simulink model "Project6"  (R2014a)
settings: Solver=ode45  StartTime=0.0  StopTime=310  RelTol=1e-3
undefined symbols (not defined in the file or in its folder): AXI4, Lite
libraries: xbsIndex_r4 x267
(part 2 of 2)

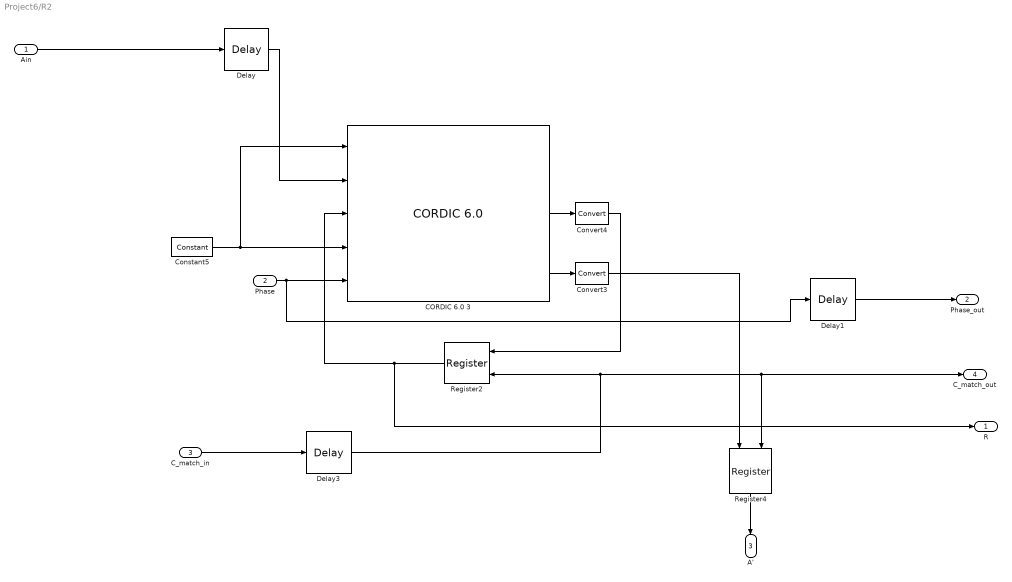
== system Project6/R2 ==
  Ain : Inport
  Phase : Inport  Port=2
  C_match_in : Inport  Port=3
  CORDIC 6.0 3 : xbsIndex_r4/CORDIC 6.0   functional_selection=Rotate  architectural_configuration=Parallel  pipelining_mode=Maximum  data_format=SignedFraction  phase_format=Radians  input_width=16  output_width=16  round_mode=Truncate  iterations=16  precision=16  compensation_scaling=LUT_based  coarse_rotation=on  aclken=off  aresetn=off  out_tready=off  cartesian_has_tuser=off  cartesian_has_tlast=off  cartesian_tuser_width=1  phase_has_tuser=off  phase_has_tlast=off  phase_tuser_width=1  out_tlast_behv=Null  flow_control=NonBlocking  optimize_goal=Performance  trim_axipin_name=on  ip_name=CORDIC  ip_version=6.0  dsptool_ready=true  ipcore_usecache=true  ipcore_useipmodelcache=true  wrapper_available=true  port_translation_map={ 'aclken' => 'en', 'aresetn' => 'rst' }  block_type=cordic_v6_0
      settings: infoedit=CORDIC 6.0
  Constant5 : xbsIndex_r4/Constant  const=1  gui_display_data_type=Boolean  arith_type=Boolean  n_bits=16  bin_pt=14  preci_type=Single  exp_width=8  frac_width=24  explicit_period=on  period=1  equ=P=C  opselect=C  inp2=PCIN>>17  opr=+  inp1=P  carry=CIN  dbl_ovrd=off  block_type=constant
  Convert3 : xbsIndex_r4/Convert  gui_display_data_type=Fixed-point  arith_type="Signed  (2's comp)"  n_bits=16  bin_pt=14  float_type=Single  exp_bits=8  fraction_bits=24  quantization=Truncate  overflow=Wrap  en=off  latency=0  pipeline=on  dbl_ovrd=off  block_type=convert
  Convert4 : xbsIndex_r4/Convert  gui_display_data_type=Fixed-point  arith_type="Signed  (2's comp)"  n_bits=16  bin_pt=14  float_type=Single  exp_bits=8  fraction_bits=24  quantization=Truncate  overflow=Wrap  en=off  latency=0  pipeline=on  dbl_ovrd=off  block_type=convert
  Delay : xbsIndex_r4/Delay  rst=off  infoeditControl=Selection of Reset will increase slice count due to use of real FFs and instead of SRLs  en=off  latency=22  reg_retiming=off  dbl_ovrd=off  block_type=delay
  Delay1 : xbsIndex_r4/Delay  rst=off  infoeditControl=Selection of Reset will increase slice count due to use of real FFs and instead of SRLs  en=off  latency=1  reg_retiming=off  dbl_ovrd=off  block_type=delay
  Delay3 : xbsIndex_r4/Delay  rst=off  infoeditControl=Selection of Reset will increase slice count due to use of real FFs and instead of SRLs  en=off  latency=1  reg_retiming=off  dbl_ovrd=off  block_type=delay
  Register2 : xbsIndex_r4/Register  init=0  rst=off  en=on  dbl_ovrd=off  block_type=register
  Register4 : xbsIndex_r4/Register  init=0  rst=off  en=on  dbl_ovrd=off  block_type=register
  R : Outport
  Phase_out : Outport  Port=2
  A' : Outport  Port=3
  C_match_out : Outport  Port=4
  wires:
  Ain/1 -> Delay/1
  Delay/1 -> CORDIC 6.0 3/2
  Convert4/1 -> Register2/1
  CORDIC 6.0 3/2 -> Convert4/1
  Register2/1 -> R/1, CORDIC 6.0 3/3
  CORDIC 6.0 3/3 -> Convert3/1
  Constant5/1 -> CORDIC 6.0 3/1, CORDIC 6.0 3/4
  Register4/1 -> A'/1
  Convert3/1 -> Register4/1
  Phase/1 -> Delay1/1, CORDIC 6.0 3/5
  Delay3/1 -> Register2/2, C_match_out/1, Register4/2
  C_match_in/1 -> Delay3/1
  Delay1/1 -> Phase_out/1

== system Project6/R22 ==
  Ain : Inport
  "C_match_in " : Inport  Port=2
  CORDIC 6.0 1 : xbsIndex_r4/CORDIC 6.0   functional_selection=Rotate  architectural_configuration=Parallel  pipelining_mode=Maximum  data_format=SignedFraction  phase_format=Radians  input_width=16  output_width=16  round_mode=Truncate  iterations=16  precision=16  compensation_scaling=LUT_based  coarse_rotation=on  aclken=off  aresetn=off  out_tready=off  cartesian_has_tuser=off  cartesian_has_tlast=off  cartesian_tuser_width=1  phase_has_tuser=off  phase_has_tlast=off  phase_tuser_width=1  out_tlast_behv=Null  flow_control=NonBlocking  optimize_goal=Performance  trim_axipin_name=on  ip_name=CORDIC  ip_version=6.0  dsptool_ready=true  ipcore_usecache=true  ipcore_useipmodelcache=true  wrapper_available=true  port_translation_map={ 'aclken' => 'en', 'aresetn' => 'rst' }  block_type=cordic_v6_0
      settings: infoedit=CORDIC 6.0
  CORDIC 6.0 2 : xbsIndex_r4/CORDIC 6.0   functional_selection=Arc_Tan  architectural_configuration=Parallel  pipelining_mode=Maximum  data_format=SignedFraction  phase_format=Radians  input_width=16  output_width=16  round_mode=Truncate  iterations=16  precision=16  compensation_scaling=No_Scale_Compensation  coarse_rotation=on  aclken=off  aresetn=off  out_tready=off  cartesian_has_tuser=off  cartesian_has_tlast=off  cartesian_tuser_width=1  phase_has_tuser=off  phase_has_tlast=off  phase_tuser_width=1  out_tlast_behv=Null  flow_control=NonBlocking  optimize_goal=Performance  trim_axipin_name=on  ip_name=CORDIC  ip_version=6.0  dsptool_ready=true  ipcore_usecache=true  ipcore_useipmodelcache=true  wrapper_available=true  port_translation_map={ 'aclken' => 'en', 'aresetn' => 'rst' }  block_type=cordic_v6_0
      settings: infoedit=CORDIC 6.0
  Constant1 : xbsIndex_r4/Constant  const=1  gui_display_data_type=Boolean  arith_type=Boolean  n_bits=16  bin_pt=14  preci_type=Single  exp_width=8  frac_width=24  explicit_period=on  period=1  equ=P=C  opselect=C  inp2=PCIN>>17  opr=+  inp1=P  carry=CIN  dbl_ovrd=off  block_type=constant
  Constant2 : xbsIndex_r4/Constant  const=1  gui_display_data_type=Boolean  arith_type=Boolean  n_bits=16  bin_pt=14  preci_type=Single  exp_width=8  frac_width=24  explicit_period=on  period=1  equ=P=C  opselect=C  inp2=PCIN>>17  opr=+  inp1=P  carry=CIN  dbl_ovrd=off  block_type=constant
  Convert1 : xbsIndex_r4/Convert  gui_display_data_type=Fixed-point  arith_type="Signed  (2's comp)"  n_bits=16  bin_pt=14  float_type=Single  exp_bits=8  fraction_bits=24  quantization=Truncate  overflow=Wrap  en=off  latency=0  pipeline=on  dbl_ovrd=off  block_type=convert
  Convert2 : xbsIndex_r4/Convert  gui_display_data_type=Fixed-point  arith_type="Signed  (2's comp)"  n_bits=16  bin_pt=14  float_type=Single  exp_bits=8  fraction_bits=24  quantization=Truncate  overflow=Wrap  en=off  latency=0  pipeline=on  dbl_ovrd=off  block_type=convert
  Delay1 : xbsIndex_r4/Delay  rst=off  infoeditControl=Selection of Reset will increase slice count due to use of real FFs and instead of SRLs  en=off  latency=1  reg_retiming=off  dbl_ovrd=off  block_type=delay
  Register : xbsIndex_r4/Register  init=0  rst=off  en=on  dbl_ovrd=off  block_type=register
  Scope1 : Scope  NumInputPorts=2
      settings: YMin=-5~-5  YMax=5~5  SaveName=ScopeData5
  Phase : Outport
  C_match_out : Outport  Port=2
  R : Outport  Port=3
  wires:
  Constant1/1 -> CORDIC 6.0 1/1, CORDIC 6.0 1/4
  Constant2/1 -> CORDIC 6.0 2/1
  Delay1/1 -> Phase/1
  CORDIC 6.0 1/2 -> Convert2/1
  CORDIC 6.0 2/2 -> Delay1/1, CORDIC 6.0 1/5
  Ain/1 -> CORDIC 6.0 2/3, Scope1/1, CORDIC 6.0 1/2
  Register/1 -> R/1, Convert1/1, CORDIC 6.0 1/3
  Convert2/1 -> Register/1
  "C_match_in "/1 -> Register/2, C_match_out/1
  Convert1/1 -> Scope1/2, CORDIC 6.0 2/2

== system Project6/R23 ==
  Ain : Inport
  Phase : Inport  Port=2
  C_match_in : Inport  Port=3
  CORDIC 6.0 3 : xbsIndex_r4/CORDIC 6.0   functional_selection=Rotate  architectural_configuration=Parallel  pipelining_mode=Maximum  data_format=SignedFraction  phase_format=Radians  input_width=16  output_width=16  round_mode=Truncate  iterations=16  precision=16  compensation_scaling=LUT_based  coarse_rotation=on  aclken=off  aresetn=off  out_tready=off  cartesian_has_tuser=off  cartesian_has_tlast=off  cartesian_tuser_width=1  phase_has_tuser=off  phase_has_tlast=off  phase_tuser_width=1  out_tlast_behv=Null  flow_control=NonBlocking  optimize_goal=Performance  trim_axipin_name=on  ip_name=CORDIC  ip_version=6.0  dsptool_ready=true  ipcore_usecache=true  ipcore_useipmodelcache=true  wrapper_available=true  port_translation_map={ 'aclken' => 'en', 'aresetn' => 'rst' }  block_type=cordic_v6_0
      settings: infoedit=CORDIC 6.0
  Constant5 : xbsIndex_r4/Constant  const=1  gui_display_data_type=Boolean  arith_type=Boolean  n_bits=16  bin_pt=14  preci_type=Single  exp_width=8  frac_width=24  explicit_period=on  period=1  equ=P=C  opselect=C  inp2=PCIN>>17  opr=+  inp1=P  carry=CIN  dbl_ovrd=off  block_type=constant
  Convert3 : xbsIndex_r4/Convert  gui_display_data_type=Fixed-point  arith_type="Signed  (2's comp)"  n_bits=16  bin_pt=14  float_type=Single  exp_bits=8  fraction_bits=24  quantization=Truncate  overflow=Wrap  en=off  latency=0  pipeline=on  dbl_ovrd=off  block_type=convert
  Convert4 : xbsIndex_r4/Convert  gui_display_data_type=Fixed-point  arith_type="Signed  (2's comp)"  n_bits=16  bin_pt=14  float_type=Single  exp_bits=8  fraction_bits=24  quantization=Truncate  overflow=Wrap  en=off  latency=0  pipeline=on  dbl_ovrd=off  block_type=convert
  Delay1 : xbsIndex_r4/Delay  rst=off  infoeditControl=Selection of Reset will increase slice count due to use of real FFs and instead of SRLs  en=off  latency=1  reg_retiming=off  dbl_ovrd=off  block_type=delay
  Delay2 : xbsIndex_r4/Delay  rst=off  infoeditControl=Selection of Reset will increase slice count due to use of real FFs and instead of SRLs  en=off  latency=22  reg_retiming=off  dbl_ovrd=off  block_type=delay
  Delay3 : xbsIndex_r4/Delay  rst=off  infoeditControl=Selection of Reset will increase slice count due to use of real FFs and instead of SRLs  en=off  latency=1  reg_retiming=off  dbl_ovrd=off  block_type=delay
  Register2 : xbsIndex_r4/Register  init=0  rst=off  en=on  dbl_ovrd=off  block_type=register
  Register4 : xbsIndex_r4/Register  init=0  rst=off  en=on  dbl_ovrd=off  block_type=register
  R : Outport
  Phase_out : Outport  Port=2
  A' : Outport  Port=3
  C_match_out : Outport  Port=4
  wires:
  CORDIC 6.0 3/2 -> Convert4/1
  Register2/1 -> R/1, CORDIC 6.0 3/3
  CORDIC 6.0 3/3 -> Convert3/1
  Constant5/1 -> CORDIC 6.0 3/1, CORDIC 6.0 3/4
  Register4/1 -> A'/1
  Convert3/1 -> Register4/1
  Delay3/1 -> Register2/2, C_match_out/1, Register4/2
  C_match_in/1 -> Delay3/1
  Delay1/1 -> Phase_out/1
  Ain/1 -> Delay2/1
  Phase/1 -> CORDIC 6.0 3/5, Delay1/1
  Delay2/1 -> CORDIC 6.0 3/2
  Convert4/1 -> Register2/1

== system Project6/R24 ==
  Ain : Inport
  Phase : Inport  Port=2
  C_match_in : Inport  Port=3
  CORDIC 6.0 3 : xbsIndex_r4/CORDIC 6.0   functional_selection=Rotate  architectural_configuration=Parallel  pipelining_mode=Maximum  data_format=SignedFraction  phase_format=Radians  input_width=16  output_width=16  round_mode=Truncate  iterations=16  precision=16  compensation_scaling=LUT_based  coarse_rotation=on  aclken=off  aresetn=off  out_tready=off  cartesian_has_tuser=off  cartesian_has_tlast=off  cartesian_tuser_width=1  phase_has_tuser=off  phase_has_tlast=off  phase_tuser_width=1  out_tlast_behv=Null  flow_control=NonBlocking  optimize_goal=Performance  trim_axipin_name=on  ip_name=CORDIC  ip_version=6.0  dsptool_ready=true  ipcore_usecache=true  ipcore_useipmodelcache=true  wrapper_available=true  port_translation_map={ 'aclken' => 'en', 'aresetn' => 'rst' }  block_type=cordic_v6_0
      settings: infoedit=CORDIC 6.0
  Constant5 : xbsIndex_r4/Constant  const=1  gui_display_data_type=Boolean  arith_type=Boolean  n_bits=16  bin_pt=14  preci_type=Single  exp_width=8  frac_width=24  explicit_period=on  period=1  equ=P=C  opselect=C  inp2=PCIN>>17  opr=+  inp1=P  carry=CIN  dbl_ovrd=off  block_type=constant
  Convert3 : xbsIndex_r4/Convert  gui_display_data_type=Fixed-point  arith_type="Signed  (2's comp)"  n_bits=16  bin_pt=14  float_type=Single  exp_bits=8  fraction_bits=24  quantization=Truncate  overflow=Wrap  en=off  latency=0  pipeline=on  dbl_ovrd=off  block_type=convert
  Convert4 : xbsIndex_r4/Convert  gui_display_data_type=Fixed-point  arith_type="Signed  (2's comp)"  n_bits=16  bin_pt=14  float_type=Single  exp_bits=8  fraction_bits=24  quantization=Truncate  overflow=Wrap  en=off  latency=0  pipeline=on  dbl_ovrd=off  block_type=convert
  Delay : xbsIndex_r4/Delay  rst=off  infoeditControl=Selection of Reset will increase slice count due to use of real FFs and instead of SRLs  en=off  latency=22  reg_retiming=off  dbl_ovrd=off  block_type=delay
  Delay1 : xbsIndex_r4/Delay  rst=off  infoeditControl=Selection of Reset will increase slice count due to use of real FFs and instead of SRLs  en=off  latency=1  reg_retiming=off  dbl_ovrd=off  block_type=delay
  Delay3 : xbsIndex_r4/Delay  rst=off  infoeditControl=Selection of Reset will increase slice count due to use of real FFs and instead of SRLs  en=off  latency=1  reg_retiming=off  dbl_ovrd=off  block_type=delay
  Register2 : xbsIndex_r4/Register  init=0  rst=off  en=on  dbl_ovrd=off  block_type=register
  Register4 : xbsIndex_r4/Register  init=0  rst=off  en=on  dbl_ovrd=off  block_type=register
  R : Outport
  Phase_out : Outport  Port=2
  A' : Outport  Port=3
  C_match_out : Outport  Port=4
  wires:
  Ain/1 -> Delay/1
  Delay/1 -> CORDIC 6.0 3/2
  Convert4/1 -> Register2/1
  CORDIC 6.0 3/2 -> Convert4/1
  Register2/1 -> R/1, CORDIC 6.0 3/3
  CORDIC 6.0 3/3 -> Convert3/1
  Constant5/1 -> CORDIC 6.0 3/1, CORDIC 6.0 3/4
  Register4/1 -> A'/1
  Convert3/1 -> Register4/1
  Phase/1 -> Delay1/1, CORDIC 6.0 3/5
  Delay3/1 -> Register2/2, C_match_out/1, Register4/2
  C_match_in/1 -> Delay3/1
  Delay1/1 -> Phase_out/1

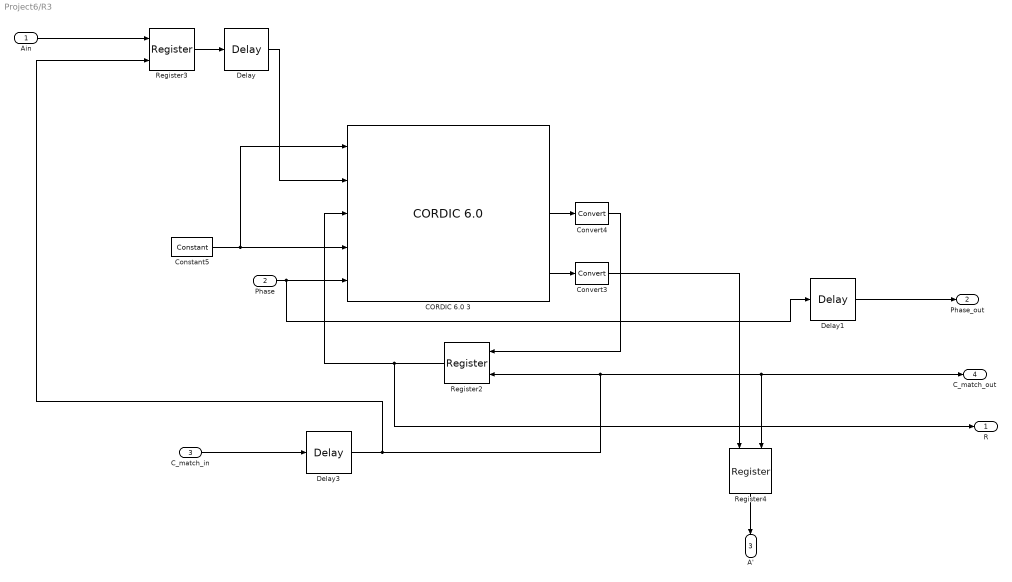
== system Project6/R3 ==
  Ain : Inport
  Phase : Inport  Port=2
  C_match_in : Inport  Port=3
  CORDIC 6.0 3 : xbsIndex_r4/CORDIC 6.0   functional_selection=Rotate  architectural_configuration=Parallel  pipelining_mode=Maximum  data_format=SignedFraction  phase_format=Radians  input_width=16  output_width=16  round_mode=Truncate  iterations=16  precision=16  compensation_scaling=LUT_based  coarse_rotation=on  aclken=off  aresetn=off  out_tready=off  cartesian_has_tuser=off  cartesian_has_tlast=off  cartesian_tuser_width=1  phase_has_tuser=off  phase_has_tlast=off  phase_tuser_width=1  out_tlast_behv=Null  flow_control=NonBlocking  optimize_goal=Performance  trim_axipin_name=on  ip_name=CORDIC  ip_version=6.0  dsptool_ready=true  ipcore_usecache=true  ipcore_useipmodelcache=true  wrapper_available=true  port_translation_map={ 'aclken' => 'en', 'aresetn' => 'rst' }  block_type=cordic_v6_0
      settings: infoedit=CORDIC 6.0
  Constant5 : xbsIndex_r4/Constant  const=1  gui_display_data_type=Boolean  arith_type=Boolean  n_bits=16  bin_pt=14  preci_type=Single  exp_width=8  frac_width=24  explicit_period=on  period=1  equ=P=C  opselect=C  inp2=PCIN>>17  opr=+  inp1=P  carry=CIN  dbl_ovrd=off  block_type=constant
  Convert3 : xbsIndex_r4/Convert  gui_display_data_type=Fixed-point  arith_type="Signed  (2's comp)"  n_bits=16  bin_pt=14  float_type=Single  exp_bits=8  fraction_bits=24  quantization=Truncate  overflow=Wrap  en=off  latency=0  pipeline=on  dbl_ovrd=off  block_type=convert
  Convert4 : xbsIndex_r4/Convert  gui_display_data_type=Fixed-point  arith_type="Signed  (2's comp)"  n_bits=16  bin_pt=14  float_type=Single  exp_bits=8  fraction_bits=24  quantization=Truncate  overflow=Wrap  en=off  latency=0  pipeline=on  dbl_ovrd=off  block_type=convert
  Delay : xbsIndex_r4/Delay  rst=off  infoeditControl=Selection of Reset will increase slice count due to use of real FFs and instead of SRLs  en=off  latency=22  reg_retiming=off  dbl_ovrd=off  block_type=delay
  Delay1 : xbsIndex_r4/Delay  rst=off  infoeditControl=Selection of Reset will increase slice count due to use of real FFs and instead of SRLs  en=off  latency=1  reg_retiming=off  dbl_ovrd=off  block_type=delay
  Delay3 : xbsIndex_r4/Delay  rst=off  infoeditControl=Selection of Reset will increase slice count due to use of real FFs and instead of SRLs  en=off  latency=1  reg_retiming=off  dbl_ovrd=off  block_type=delay
  Register2 : xbsIndex_r4/Register  init=0  rst=off  en=on  dbl_ovrd=off  block_type=register
  Register3 : xbsIndex_r4/Register  init=0  rst=off  en=on  dbl_ovrd=off  block_type=register
  Register4 : xbsIndex_r4/Register  init=0  rst=off  en=on  dbl_ovrd=off  block_type=register
  R : Outport
  Phase_out : Outport  Port=2
  A' : Outport  Port=3
  C_match_out : Outport  Port=4
  wires:
  Register3/1 -> Delay/1
  Ain/1 -> Register3/1
  Delay/1 -> CORDIC 6.0 3/2
  Convert4/1 -> Register2/1
  CORDIC 6.0 3/2 -> Convert4/1
  Register2/1 -> R/1, CORDIC 6.0 3/3
  CORDIC 6.0 3/3 -> Convert3/1
  Constant5/1 -> CORDIC 6.0 3/1, CORDIC 6.0 3/4
  Register4/1 -> A'/1
  Convert3/1 -> Register4/1
  Phase/1 -> Delay1/1, CORDIC 6.0 3/5
  Delay3/1 -> Register3/2, Register2/2, C_match_out/1, Register4/2
  C_match_in/1 -> Delay3/1
  Delay1/1 -> Phase_out/1

== system Project6/R33 ==
  Ain : Inport
  "C_match_in " : Inport  Port=2
  CORDIC 6.0 1 : xbsIndex_r4/CORDIC 6.0   functional_selection=Rotate  architectural_configuration=Parallel  pipelining_mode=Maximum  data_format=SignedFraction  phase_format=Radians  input_width=16  output_width=16  round_mode=Truncate  iterations=16  precision=16  compensation_scaling=LUT_based  coarse_rotation=on  aclken=off  aresetn=off  out_tready=off  cartesian_has_tuser=off  cartesian_has_tlast=off  cartesian_tuser_width=1  phase_has_tuser=off  phase_has_tlast=off  phase_tuser_width=1  out_tlast_behv=Null  flow_control=NonBlocking  optimize_goal=Performance  trim_axipin_name=on  ip_name=CORDIC  ip_version=6.0  dsptool_ready=true  ipcore_usecache=true  ipcore_useipmodelcache=true  wrapper_available=true  port_translation_map={ 'aclken' => 'en', 'aresetn' => 'rst' }  block_type=cordic_v6_0
      settings: infoedit=CORDIC 6.0
  CORDIC 6.0 2 : xbsIndex_r4/CORDIC 6.0   functional_selection=Arc_Tan  architectural_configuration=Parallel  pipelining_mode=Maximum  data_format=SignedFraction  phase_format=Radians  input_width=16  output_width=16  round_mode=Truncate  iterations=16  precision=16  compensation_scaling=No_Scale_Compensation  coarse_rotation=on  aclken=off  aresetn=off  out_tready=off  cartesian_has_tuser=off  cartesian_has_tlast=off  cartesian_tuser_width=1  phase_has_tuser=off  phase_has_tlast=off  phase_tuser_width=1  out_tlast_behv=Null  flow_control=NonBlocking  optimize_goal=Performance  trim_axipin_name=on  ip_name=CORDIC  ip_version=6.0  dsptool_ready=true  ipcore_usecache=true  ipcore_useipmodelcache=true  wrapper_available=true  port_translation_map={ 'aclken' => 'en', 'aresetn' => 'rst' }  block_type=cordic_v6_0
      settings: infoedit=CORDIC 6.0
  Constant1 : xbsIndex_r4/Constant  const=1  gui_display_data_type=Boolean  arith_type=Boolean  n_bits=16  bin_pt=14  preci_type=Single  exp_width=8  frac_width=24  explicit_period=on  period=1  equ=P=C  opselect=C  inp2=PCIN>>17  opr=+  inp1=P  carry=CIN  dbl_ovrd=off  block_type=constant
  Constant2 : xbsIndex_r4/Constant  const=1  gui_display_data_type=Boolean  arith_type=Boolean  n_bits=16  bin_pt=14  preci_type=Single  exp_width=8  frac_width=24  explicit_period=on  period=1  equ=P=C  opselect=C  inp2=PCIN>>17  opr=+  inp1=P  carry=CIN  dbl_ovrd=off  block_type=constant
  Convert1 : xbsIndex_r4/Convert  gui_display_data_type=Fixed-point  arith_type="Signed  (2's comp)"  n_bits=16  bin_pt=14  float_type=Single  exp_bits=8  fraction_bits=24  quantization=Truncate  overflow=Wrap  en=off  latency=0  pipeline=on  dbl_ovrd=off  block_type=convert
  Convert2 : xbsIndex_r4/Convert  gui_display_data_type=Fixed-point  arith_type="Signed  (2's comp)"  n_bits=16  bin_pt=14  float_type=Single  exp_bits=8  fraction_bits=24  quantization=Truncate  overflow=Wrap  en=off  latency=0  pipeline=on  dbl_ovrd=off  block_type=convert
  Delay1 : xbsIndex_r4/Delay  rst=off  infoeditControl=Selection of Reset will increase slice count due to use of real FFs and instead of SRLs  en=off  latency=1  reg_retiming=off  dbl_ovrd=off  block_type=delay
  Register : xbsIndex_r4/Register  init=0  rst=off  en=on  dbl_ovrd=off  block_type=register
  Phase : Outport
  C_match_out : Outport  Port=2
  R : Outport  Port=3
  wires:
  Constant1/1 -> CORDIC 6.0 1/1, CORDIC 6.0 1/4
  Constant2/1 -> CORDIC 6.0 2/1
  Delay1/1 -> Phase/1
  CORDIC 6.0 1/2 -> Convert2/1
  CORDIC 6.0 2/2 -> Delay1/1, CORDIC 6.0 1/5
  Ain/1 -> CORDIC 6.0 2/3, CORDIC 6.0 1/2
  Convert1/1 -> CORDIC 6.0 2/2
  Register/1 -> R/1, Convert1/1, CORDIC 6.0 1/3
  Convert2/1 -> Register/1
  "C_match_in "/1 -> Register/2, C_match_out/1

== system Project6/R34 ==
  Ain : Inport
  Phase : Inport  Port=2
  C_match_in : Inport  Port=3
  CORDIC 6.0 3 : xbsIndex_r4/CORDIC 6.0   functional_selection=Rotate  architectural_configuration=Parallel  pipelining_mode=Maximum  data_format=SignedFraction  phase_format=Radians  input_width=16  output_width=16  round_mode=Truncate  iterations=16  precision=16  compensation_scaling=LUT_based  coarse_rotation=on  aclken=off  aresetn=off  out_tready=off  cartesian_has_tuser=off  cartesian_has_tlast=off  cartesian_tuser_width=1  phase_has_tuser=off  phase_has_tlast=off  phase_tuser_width=1  out_tlast_behv=Null  flow_control=NonBlocking  optimize_goal=Performance  trim_axipin_name=on  ip_name=CORDIC  ip_version=6.0  dsptool_ready=true  ipcore_usecache=true  ipcore_useipmodelcache=true  wrapper_available=true  port_translation_map={ 'aclken' => 'en', 'aresetn' => 'rst' }  block_type=cordic_v6_0
      settings: infoedit=CORDIC 6.0
  Constant5 : xbsIndex_r4/Constant  const=1  gui_display_data_type=Boolean  arith_type=Boolean  n_bits=16  bin_pt=14  preci_type=Single  exp_width=8  frac_width=24  explicit_period=on  period=1  equ=P=C  opselect=C  inp2=PCIN>>17  opr=+  inp1=P  carry=CIN  dbl_ovrd=off  block_type=constant
  Convert3 : xbsIndex_r4/Convert  gui_display_data_type=Fixed-point  arith_type="Signed  (2's comp)"  n_bits=16  bin_pt=14  float_type=Single  exp_bits=8  fraction_bits=24  quantization=Truncate  overflow=Wrap  en=off  latency=0  pipeline=on  dbl_ovrd=off  block_type=convert
  Convert4 : xbsIndex_r4/Convert  gui_display_data_type=Fixed-point  arith_type="Signed  (2's comp)"  n_bits=16  bin_pt=14  float_type=Single  exp_bits=8  fraction_bits=24  quantization=Truncate  overflow=Wrap  en=off  latency=0  pipeline=on  dbl_ovrd=off  block_type=convert
  Delay : xbsIndex_r4/Delay  rst=off  infoeditControl=Selection of Reset will increase slice count due to use of real FFs and instead of SRLs  en=off  latency=22  reg_retiming=off  dbl_ovrd=off  block_type=delay
  Delay1 : xbsIndex_r4/Delay  rst=off  infoeditControl=Selection of Reset will increase slice count due to use of real FFs and instead of SRLs  en=off  latency=1  reg_retiming=off  dbl_ovrd=off  block_type=delay
  Delay3 : xbsIndex_r4/Delay  rst=off  infoeditControl=Selection of Reset will increase slice count due to use of real FFs and instead of SRLs  en=off  latency=1  reg_retiming=off  dbl_ovrd=off  block_type=delay
  Register2 : xbsIndex_r4/Register  init=0  rst=off  en=on  dbl_ovrd=off  block_type=register
  Register4 : xbsIndex_r4/Register  init=0  rst=off  en=on  dbl_ovrd=off  block_type=register
  R : Outport
  Phase_out : Outport  Port=2
  A' : Outport  Port=3
  C_match_out : Outport  Port=4
  wires:
  Ain/1 -> Delay/1
  Delay/1 -> CORDIC 6.0 3/2
  Convert4/1 -> Register2/1
  CORDIC 6.0 3/2 -> Convert4/1
  Register2/1 -> R/1, CORDIC 6.0 3/3
  CORDIC 6.0 3/3 -> Convert3/1
  Constant5/1 -> CORDIC 6.0 3/1, CORDIC 6.0 3/4
  Register4/1 -> A'/1
  Convert3/1 -> Register4/1
  Phase/1 -> Delay1/1, CORDIC 6.0 3/5
  Delay3/1 -> Register2/2, C_match_out/1, Register4/2
  C_match_in/1 -> Delay3/1
  Delay1/1 -> Phase_out/1

== system Project6/R4 ==
  Ain : Inport
  Phase : Inport  Port=2
  C_match_in : Inport  Port=3
  CORDIC 6.0 3 : xbsIndex_r4/CORDIC 6.0   functional_selection=Rotate  architectural_configuration=Parallel  pipelining_mode=Maximum  data_format=SignedFraction  phase_format=Radians  input_width=16  output_width=16  round_mode=Truncate  iterations=16  precision=16  compensation_scaling=LUT_based  coarse_rotation=on  aclken=off  aresetn=off  out_tready=off  cartesian_has_tuser=off  cartesian_has_tlast=off  cartesian_tuser_width=1  phase_has_tuser=off  phase_has_tlast=off  phase_tuser_width=1  out_tlast_behv=Null  flow_control=NonBlocking  optimize_goal=Performance  trim_axipin_name=on  ip_name=CORDIC  ip_version=6.0  dsptool_ready=true  ipcore_usecache=true  ipcore_useipmodelcache=true  wrapper_available=true  port_translation_map={ 'aclken' => 'en', 'aresetn' => 'rst' }  block_type=cordic_v6_0
      settings: infoedit=CORDIC 6.0
  Constant5 : xbsIndex_r4/Constant  const=1  gui_display_data_type=Boolean  arith_type=Boolean  n_bits=16  bin_pt=14  preci_type=Single  exp_width=8  frac_width=24  explicit_period=on  period=1  equ=P=C  opselect=C  inp2=PCIN>>17  opr=+  inp1=P  carry=CIN  dbl_ovrd=off  block_type=constant
  Convert3 : xbsIndex_r4/Convert  gui_display_data_type=Fixed-point  arith_type="Signed  (2's comp)"  n_bits=16  bin_pt=14  float_type=Single  exp_bits=8  fraction_bits=24  quantization=Truncate  overflow=Wrap  en=off  latency=0  pipeline=on  dbl_ovrd=off  block_type=convert
  Convert4 : xbsIndex_r4/Convert  gui_display_data_type=Fixed-point  arith_type="Signed  (2's comp)"  n_bits=16  bin_pt=14  float_type=Single  exp_bits=8  fraction_bits=24  quantization=Truncate  overflow=Wrap  en=off  latency=0  pipeline=on  dbl_ovrd=off  block_type=convert
  Delay : xbsIndex_r4/Delay  rst=off  infoeditControl=Selection of Reset will increase slice count due to use of real FFs and instead of SRLs  en=off  latency=22  reg_retiming=off  dbl_ovrd=off  block_type=delay
  Delay1 : xbsIndex_r4/Delay  rst=off  infoeditControl=Selection of Reset will increase slice count due to use of real FFs and instead of SRLs  en=off  latency=1  reg_retiming=off  dbl_ovrd=off  block_type=delay
  Delay3 : xbsIndex_r4/Delay  rst=off  infoeditControl=Selection of Reset will increase slice count due to use of real FFs and instead of SRLs  en=off  latency=1  reg_retiming=off  dbl_ovrd=off  block_type=delay
  Register2 : xbsIndex_r4/Register  init=0  rst=off  en=on  dbl_ovrd=off  block_type=register
  Register4 : xbsIndex_r4/Register  init=0  rst=off  en=on  dbl_ovrd=off  block_type=register
  R : Outport
  Phase_out : Outport  Port=2
  A' : Outport  Port=3
  C_match_out : Outport  Port=4
  wires:
  Ain/1 -> Delay/1
  Delay/1 -> CORDIC 6.0 3/2
  Convert4/1 -> Register2/1
  CORDIC 6.0 3/2 -> Convert4/1
  Register2/1 -> R/1, CORDIC 6.0 3/3
  CORDIC 6.0 3/3 -> Convert3/1
  Constant5/1 -> CORDIC 6.0 3/1, CORDIC 6.0 3/4
  Register4/1 -> A'/1
  Convert3/1 -> Register4/1
  Phase/1 -> Delay1/1, CORDIC 6.0 3/5
  Delay3/1 -> Register2/2, C_match_out/1, Register4/2
  C_match_in/1 -> Delay3/1
  Delay1/1 -> Phase_out/1

== system Project6/R5 ==
  Ain : Inport
  Phase : Inport  Port=2
  C_match_in : Inport  Port=3
  CORDIC 6.0 3 : xbsIndex_r4/CORDIC 6.0   functional_selection=Rotate  architectural_configuration=Parallel  pipelining_mode=Maximum  data_format=SignedFraction  phase_format=Radians  input_width=16  output_width=16  round_mode=Truncate  iterations=16  precision=16  compensation_scaling=LUT_based  coarse_rotation=on  aclken=off  aresetn=off  out_tready=off  cartesian_has_tuser=off  cartesian_has_tlast=off  cartesian_tuser_width=1  phase_has_tuser=off  phase_has_tlast=off  phase_tuser_width=1  out_tlast_behv=Null  flow_control=NonBlocking  optimize_goal=Performance  trim_axipin_name=on  ip_name=CORDIC  ip_version=6.0  dsptool_ready=true  ipcore_usecache=true  ipcore_useipmodelcache=true  wrapper_available=true  port_translation_map={ 'aclken' => 'en', 'aresetn' => 'rst' }  block_type=cordic_v6_0
      settings: infoedit=CORDIC 6.0
  Constant5 : xbsIndex_r4/Constant  const=1  gui_display_data_type=Boolean  arith_type=Boolean  n_bits=16  bin_pt=14  preci_type=Single  exp_width=8  frac_width=24  explicit_period=on  period=1  equ=P=C  opselect=C  inp2=PCIN>>17  opr=+  inp1=P  carry=CIN  dbl_ovrd=off  block_type=constant
  Convert3 : xbsIndex_r4/Convert  gui_display_data_type=Fixed-point  arith_type="Signed  (2's comp)"  n_bits=16  bin_pt=14  float_type=Single  exp_bits=8  fraction_bits=24  quantization=Truncate  overflow=Wrap  en=off  latency=0  pipeline=on  dbl_ovrd=off  block_type=convert
  Convert4 : xbsIndex_r4/Convert  gui_display_data_type=Fixed-point  arith_type="Signed  (2's comp)"  n_bits=16  bin_pt=14  float_type=Single  exp_bits=8  fraction_bits=24  quantization=Truncate  overflow=Wrap  en=off  latency=0  pipeline=on  dbl_ovrd=off  block_type=convert
  Delay : xbsIndex_r4/Delay  rst=off  infoeditControl=Selection of Reset will increase slice count due to use of real FFs and instead of SRLs  en=off  latency=22  reg_retiming=off  dbl_ovrd=off  block_type=delay
  Delay1 : xbsIndex_r4/Delay  rst=off  infoeditControl=Selection of Reset will increase slice count due to use of real FFs and instead of SRLs  en=off  latency=1  reg_retiming=off  dbl_ovrd=off  block_type=delay
  Delay3 : xbsIndex_r4/Delay  rst=off  infoeditControl=Selection of Reset will increase slice count due to use of real FFs and instead of SRLs  en=off  latency=1  reg_retiming=off  dbl_ovrd=off  block_type=delay
  Register2 : xbsIndex_r4/Register  init=0  rst=off  en=on  dbl_ovrd=off  block_type=register
  Register4 : xbsIndex_r4/Register  init=0  rst=off  en=on  dbl_ovrd=off  block_type=register
  R : Outport
  Phase_out : Outport  Port=2
  A' : Outport  Port=3
  C_match_out : Outport  Port=4
  wires:
  Ain/1 -> Delay/1
  Delay/1 -> CORDIC 6.0 3/2
  Convert4/1 -> Register2/1
  CORDIC 6.0 3/2 -> Convert4/1
  Register2/1 -> R/1, CORDIC 6.0 3/3
  CORDIC 6.0 3/3 -> Convert3/1
  Constant5/1 -> CORDIC 6.0 3/1, CORDIC 6.0 3/4
  Register4/1 -> A'/1
  Convert3/1 -> Register4/1
  Phase/1 -> Delay1/1, CORDIC 6.0 3/5
  Delay3/1 -> Register2/2, C_match_out/1, Register4/2
  C_match_in/1 -> Delay3/1
  Delay1/1 -> Phase_out/1

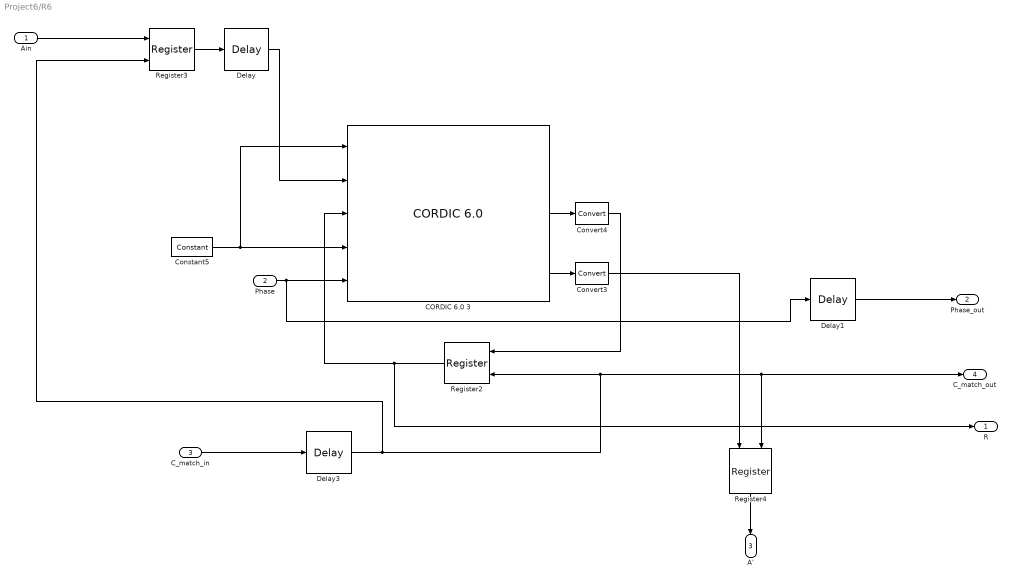
== system Project6/R6 ==
  Ain : Inport
  Phase : Inport  Port=2
  C_match_in : Inport  Port=3
  CORDIC 6.0 3 : xbsIndex_r4/CORDIC 6.0   functional_selection=Rotate  architectural_configuration=Parallel  pipelining_mode=Maximum  data_format=SignedFraction  phase_format=Radians  input_width=16  output_width=16  round_mode=Truncate  iterations=16  precision=16  compensation_scaling=LUT_based  coarse_rotation=on  aclken=off  aresetn=off  out_tready=off  cartesian_has_tuser=off  cartesian_has_tlast=off  cartesian_tuser_width=1  phase_has_tuser=off  phase_has_tlast=off  phase_tuser_width=1  out_tlast_behv=Null  flow_control=NonBlocking  optimize_goal=Performance  trim_axipin_name=on  ip_name=CORDIC  ip_version=6.0  dsptool_ready=true  ipcore_usecache=true  ipcore_useipmodelcache=true  wrapper_available=true  port_translation_map={ 'aclken' => 'en', 'aresetn' => 'rst' }  block_type=cordic_v6_0
      settings: infoedit=CORDIC 6.0
  Constant5 : xbsIndex_r4/Constant  const=1  gui_display_data_type=Boolean  arith_type=Boolean  n_bits=16  bin_pt=14  preci_type=Single  exp_width=8  frac_width=24  explicit_period=on  period=1  equ=P=C  opselect=C  inp2=PCIN>>17  opr=+  inp1=P  carry=CIN  dbl_ovrd=off  block_type=constant
  Convert3 : xbsIndex_r4/Convert  gui_display_data_type=Fixed-point  arith_type="Signed  (2's comp)"  n_bits=16  bin_pt=14  float_type=Single  exp_bits=8  fraction_bits=24  quantization=Truncate  overflow=Wrap  en=off  latency=0  pipeline=on  dbl_ovrd=off  block_type=convert
  Convert4 : xbsIndex_r4/Convert  gui_display_data_type=Fixed-point  arith_type="Signed  (2's comp)"  n_bits=16  bin_pt=14  float_type=Single  exp_bits=8  fraction_bits=24  quantization=Truncate  overflow=Wrap  en=off  latency=0  pipeline=on  dbl_ovrd=off  block_type=convert
  Delay : xbsIndex_r4/Delay  rst=off  infoeditControl=Selection of Reset will increase slice count due to use of real FFs and instead of SRLs  en=off  latency=22  reg_retiming=off  dbl_ovrd=off  block_type=delay
  Delay1 : xbsIndex_r4/Delay  rst=off  infoeditControl=Selection of Reset will increase slice count due to use of real FFs and instead of SRLs  en=off  latency=1  reg_retiming=off  dbl_ovrd=off  block_type=delay
  Delay3 : xbsIndex_r4/Delay  rst=off  infoeditControl=Selection of Reset will increase slice count due to use of real FFs and instead of SRLs  en=off  latency=1  reg_retiming=off  dbl_ovrd=off  block_type=delay
  Register2 : xbsIndex_r4/Register  init=0  rst=off  en=on  dbl_ovrd=off  block_type=register
  Register3 : xbsIndex_r4/Register  init=0  rst=off  en=on  dbl_ovrd=off  block_type=register
  Register4 : xbsIndex_r4/Register  init=0  rst=off  en=on  dbl_ovrd=off  block_type=register
  R : Outport
  Phase_out : Outport  Port=2
  A' : Outport  Port=3
  C_match_out : Outport  Port=4
  wires:
  Register3/1 -> Delay/1
  Ain/1 -> Register3/1
  Delay/1 -> CORDIC 6.0 3/2
  Convert4/1 -> Register2/1
  CORDIC 6.0 3/2 -> Convert4/1
  Register2/1 -> R/1, CORDIC 6.0 3/3
  CORDIC 6.0 3/3 -> Convert3/1
  Constant5/1 -> CORDIC 6.0 3/1, CORDIC 6.0 3/4
  Register4/1 -> A'/1
  Convert3/1 -> Register4/1
  Phase/1 -> Delay1/1, CORDIC 6.0 3/5
  Delay3/1 -> Register3/2, Register2/2, C_match_out/1, Register4/2
  C_match_in/1 -> Delay3/1
  Delay1/1 -> Phase_out/1

== system Project6/R7 ==
  Ain : Inport
  Phase : Inport  Port=2
  C_match_in : Inport  Port=3
  CORDIC 6.0 3 : xbsIndex_r4/CORDIC 6.0   functional_selection=Rotate  architectural_configuration=Parallel  pipelining_mode=Maximum  data_format=SignedFraction  phase_format=Radians  input_width=16  output_width=16  round_mode=Truncate  iterations=16  precision=16  compensation_scaling=LUT_based  coarse_rotation=on  aclken=off  aresetn=off  out_tready=off  cartesian_has_tuser=off  cartesian_has_tlast=off  cartesian_tuser_width=1  phase_has_tuser=off  phase_has_tlast=off  phase_tuser_width=1  out_tlast_behv=Null  flow_control=NonBlocking  optimize_goal=Performance  trim_axipin_name=on  ip_name=CORDIC  ip_version=6.0  dsptool_ready=true  ipcore_usecache=true  ipcore_useipmodelcache=true  wrapper_available=true  port_translation_map={ 'aclken' => 'en', 'aresetn' => 'rst' }  block_type=cordic_v6_0
      settings: infoedit=CORDIC 6.0
  Constant5 : xbsIndex_r4/Constant  const=1  gui_display_data_type=Boolean  arith_type=Boolean  n_bits=16  bin_pt=14  preci_type=Single  exp_width=8  frac_width=24  explicit_period=on  period=1  equ=P=C  opselect=C  inp2=PCIN>>17  opr=+  inp1=P  carry=CIN  dbl_ovrd=off  block_type=constant
  Convert3 : xbsIndex_r4/Convert  gui_display_data_type=Fixed-point  arith_type="Signed  (2's comp)"  n_bits=16  bin_pt=14  float_type=Single  exp_bits=8  fraction_bits=24  quantization=Truncate  overflow=Wrap  en=off  latency=0  pipeline=on  dbl_ovrd=off  block_type=convert
  Convert4 : xbsIndex_r4/Convert  gui_display_data_type=Fixed-point  arith_type="Signed  (2's comp)"  n_bits=16  bin_pt=14  float_type=Single  exp_bits=8  fraction_bits=24  quantization=Truncate  overflow=Wrap  en=off  latency=0  pipeline=on  dbl_ovrd=off  block_type=convert
  Delay : xbsIndex_r4/Delay  rst=off  infoeditControl=Selection of Reset will increase slice count due to use of real FFs and instead of SRLs  en=off  latency=22  reg_retiming=off  dbl_ovrd=off  block_type=delay
  Delay1 : xbsIndex_r4/Delay  rst=off  infoeditControl=Selection of Reset will increase slice count due to use of real FFs and instead of SRLs  en=off  latency=1  reg_retiming=off  dbl_ovrd=off  block_type=delay
  Delay3 : xbsIndex_r4/Delay  rst=off  infoeditControl=Selection of Reset will increase slice count due to use of real FFs and instead of SRLs  en=off  latency=1  reg_retiming=off  dbl_ovrd=off  block_type=delay
  Register2 : xbsIndex_r4/Register  init=0  rst=off  en=on  dbl_ovrd=off  block_type=register
  Register4 : xbsIndex_r4/Register  init=0  rst=off  en=on  dbl_ovrd=off  block_type=register
  R : Outport
  Phase_out : Outport  Port=2
  A' : Outport  Port=3
  C_match_out : Outport  Port=4
  wires:
  Ain/1 -> Delay/1
  Delay/1 -> CORDIC 6.0 3/2
  Convert4/1 -> Register2/1
  CORDIC 6.0 3/2 -> Convert4/1
  Register2/1 -> R/1, CORDIC 6.0 3/3
  CORDIC 6.0 3/3 -> Convert3/1
  Constant5/1 -> CORDIC 6.0 3/1, CORDIC 6.0 3/4
  Register4/1 -> A'/1
  Convert3/1 -> Register4/1
  Phase/1 -> Delay1/1, CORDIC 6.0 3/5
  Delay3/1 -> Register2/2, C_match_out/1, Register4/2
  C_match_in/1 -> Delay3/1
  Delay1/1 -> Phase_out/1

== system Project6/R8 ==
  Ain : Inport
  Phase : Inport  Port=2
  C_match_in : Inport  Port=3
  CORDIC 6.0 3 : xbsIndex_r4/CORDIC 6.0   functional_selection=Rotate  architectural_configuration=Parallel  pipelining_mode=Maximum  data_format=SignedFraction  phase_format=Radians  input_width=16  output_width=16  round_mode=Truncate  iterations=16  precision=16  compensation_scaling=LUT_based  coarse_rotation=on  aclken=off  aresetn=off  out_tready=off  cartesian_has_tuser=off  cartesian_has_tlast=off  cartesian_tuser_width=1  phase_has_tuser=off  phase_has_tlast=off  phase_tuser_width=1  out_tlast_behv=Null  flow_control=NonBlocking  optimize_goal=Performance  trim_axipin_name=on  ip_name=CORDIC  ip_version=6.0  dsptool_ready=true  ipcore_usecache=true  ipcore_useipmodelcache=true  wrapper_available=true  port_translation_map={ 'aclken' => 'en', 'aresetn' => 'rst' }  block_type=cordic_v6_0
      settings: infoedit=CORDIC 6.0
  Constant5 : xbsIndex_r4/Constant  const=1  gui_display_data_type=Boolean  arith_type=Boolean  n_bits=16  bin_pt=14  preci_type=Single  exp_width=8  frac_width=24  explicit_period=on  period=1  equ=P=C  opselect=C  inp2=PCIN>>17  opr=+  inp1=P  carry=CIN  dbl_ovrd=off  block_type=constant
  Convert3 : xbsIndex_r4/Convert  gui_display_data_type=Fixed-point  arith_type="Signed  (2's comp)"  n_bits=16  bin_pt=14  float_type=Single  exp_bits=8  fraction_bits=24  quantization=Truncate  overflow=Wrap  en=off  latency=0  pipeline=on  dbl_ovrd=off  block_type=convert
  Convert4 : xbsIndex_r4/Convert  gui_display_data_type=Fixed-point  arith_type="Signed  (2's comp)"  n_bits=16  bin_pt=14  float_type=Single  exp_bits=8  fraction_bits=24  quantization=Truncate  overflow=Wrap  en=off  latency=0  pipeline=on  dbl_ovrd=off  block_type=convert
  Delay : xbsIndex_r4/Delay  rst=off  infoeditControl=Selection of Reset will increase slice count due to use of real FFs and instead of SRLs  en=off  latency=22  reg_retiming=off  dbl_ovrd=off  block_type=delay
  Delay1 : xbsIndex_r4/Delay  rst=off  infoeditControl=Selection of Reset will increase slice count due to use of real FFs and instead of SRLs  en=off  latency=1  reg_retiming=off  dbl_ovrd=off  block_type=delay
  Delay3 : xbsIndex_r4/Delay  rst=off  infoeditControl=Selection of Reset will increase slice count due to use of real FFs and instead of SRLs  en=off  latency=1  reg_retiming=off  dbl_ovrd=off  block_type=delay
  Register2 : xbsIndex_r4/Register  init=0  rst=off  en=on  dbl_ovrd=off  block_type=register
  Register4 : xbsIndex_r4/Register  init=0  rst=off  en=on  dbl_ovrd=off  block_type=register
  R : Outport
  Phase_out : Outport  Port=2
  A' : Outport  Port=3
  C_match_out : Outport  Port=4
  wires:
  Ain/1 -> Delay/1
  Delay/1 -> CORDIC 6.0 3/2
  Convert4/1 -> Register2/1
  CORDIC 6.0 3/2 -> Convert4/1
  Register2/1 -> R/1, CORDIC 6.0 3/3
  CORDIC 6.0 3/3 -> Convert3/1
  Constant5/1 -> CORDIC 6.0 3/1, CORDIC 6.0 3/4
  Register4/1 -> A'/1
  Convert3/1 -> Register4/1
  Phase/1 -> Delay1/1, CORDIC 6.0 3/5
  Delay3/1 -> Register2/2, C_match_out/1, Register4/2
  C_match_in/1 -> Delay3/1
  Delay1/1 -> Phase_out/1

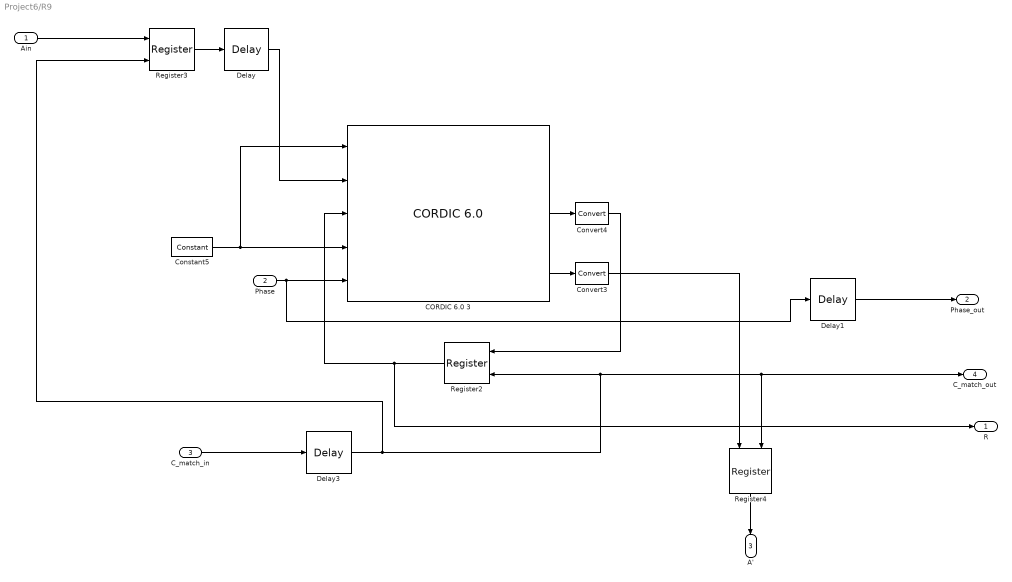
== system Project6/R9 ==
  Ain : Inport
  Phase : Inport  Port=2
  C_match_in : Inport  Port=3
  CORDIC 6.0 3 : xbsIndex_r4/CORDIC 6.0   functional_selection=Rotate  architectural_configuration=Parallel  pipelining_mode=Maximum  data_format=SignedFraction  phase_format=Radians  input_width=16  output_width=16  round_mode=Truncate  iterations=16  precision=16  compensation_scaling=LUT_based  coarse_rotation=on  aclken=off  aresetn=off  out_tready=off  cartesian_has_tuser=off  cartesian_has_tlast=off  cartesian_tuser_width=1  phase_has_tuser=off  phase_has_tlast=off  phase_tuser_width=1  out_tlast_behv=Null  flow_control=NonBlocking  optimize_goal=Performance  trim_axipin_name=on  ip_name=CORDIC  ip_version=6.0  dsptool_ready=true  ipcore_usecache=true  ipcore_useipmodelcache=true  wrapper_available=true  port_translation_map={ 'aclken' => 'en', 'aresetn' => 'rst' }  block_type=cordic_v6_0
      settings: infoedit=CORDIC 6.0
  Constant5 : xbsIndex_r4/Constant  const=1  gui_display_data_type=Boolean  arith_type=Boolean  n_bits=16  bin_pt=14  preci_type=Single  exp_width=8  frac_width=24  explicit_period=on  period=1  equ=P=C  opselect=C  inp2=PCIN>>17  opr=+  inp1=P  carry=CIN  dbl_ovrd=off  block_type=constant
  Convert3 : xbsIndex_r4/Convert  gui_display_data_type=Fixed-point  arith_type="Signed  (2's comp)"  n_bits=16  bin_pt=14  float_type=Single  exp_bits=8  fraction_bits=24  quantization=Truncate  overflow=Wrap  en=off  latency=0  pipeline=on  dbl_ovrd=off  block_type=convert
  Convert4 : xbsIndex_r4/Convert  gui_display_data_type=Fixed-point  arith_type="Signed  (2's comp)"  n_bits=16  bin_pt=14  float_type=Single  exp_bits=8  fraction_bits=24  quantization=Truncate  overflow=Wrap  en=off  latency=0  pipeline=on  dbl_ovrd=off  block_type=convert
  Delay : xbsIndex_r4/Delay  rst=off  infoeditControl=Selection of Reset will increase slice count due to use of real FFs and instead of SRLs  en=off  latency=22  reg_retiming=off  dbl_ovrd=off  block_type=delay
  Delay1 : xbsIndex_r4/Delay  rst=off  infoeditControl=Selection of Reset will increase slice count due to use of real FFs and instead of SRLs  en=off  latency=1  reg_retiming=off  dbl_ovrd=off  block_type=delay
  Delay3 : xbsIndex_r4/Delay  rst=off  infoeditControl=Selection of Reset will increase slice count due to use of real FFs and instead of SRLs  en=off  latency=1  reg_retiming=off  dbl_ovrd=off  block_type=delay
  Register2 : xbsIndex_r4/Register  init=0  rst=off  en=on  dbl_ovrd=off  block_type=register
  Register3 : xbsIndex_r4/Register  init=0  rst=off  en=on  dbl_ovrd=off  block_type=register
  Register4 : xbsIndex_r4/Register  init=0  rst=off  en=on  dbl_ovrd=off  block_type=register
  R : Outport
  Phase_out : Outport  Port=2
  A' : Outport  Port=3
  C_match_out : Outport  Port=4
  wires:
  Register3/1 -> Delay/1
  Ain/1 -> Register3/1
  Delay/1 -> CORDIC 6.0 3/2
  Convert4/1 -> Register2/1
  CORDIC 6.0 3/2 -> Convert4/1
  Register2/1 -> R/1, CORDIC 6.0 3/3
  CORDIC 6.0 3/3 -> Convert3/1
  Constant5/1 -> CORDIC 6.0 3/1, CORDIC 6.0 3/4
  Register4/1 -> A'/1
  Convert3/1 -> Register4/1
  Phase/1 -> Delay1/1, CORDIC 6.0 3/5
  Delay3/1 -> Register3/2, Register2/2, C_match_out/1, Register4/2
  C_match_in/1 -> Delay3/1
  Delay1/1 -> Phase_out/1
